simulink model "air_m0c"  (R2022b)
settings: Solver=FixedStepAuto  StartTime=0.0  StopTime=10.0  FixedStep=0.001  RelTol=1e-3  EnableMultiTasking=on
values from neighbouring files (symbols this model uses):
  dev = abs(cand(k) - cand(k - 1))    [m3_check_execution.m]
undefined symbols (not defined in the file or in its folder): Main, pwm_output0
libraries: simulink x1, px4lib x1, px4Sensorslib x1, shared6dof x1, sharedtransform x1
settings Model: ExtModeTrigDuration=10  Creator=admin  LastModifiedBy=10444
settings SolverCC: AlgebraicLoopSolver=TrustRegion  PositivePriorityOrder=on  AutoInsertRateTranBlk=on  MaxZcPerStep=1
settings OptimizationCC: EnhancedBackFolding=on  PassReuseOutputArgsAs=Individual arguments  ZeroExternalMemoryAtStartup=off  ZeroInternalMemoryAtStartup=off  MaxStackSize=64  OptimizeBlockOrder=speed  DifferentSizesBufferReuse=on  OptimizationCustomize=off  EfficientTunableParamExpr=on
settings DebuggingCC: ParameterTunabilityLossMsg=error  UnconnectedInputMsg=warning  UnconnectedOutputMsg=warning  UnconnectedLineMsg=warning  SymbolicDimsDataTypeCodeGenerationDiagnostic=none  SFMachineParentedDataDiag=warning
settings HardwareCC: ProdBitPerPointer=32  ProdBitPerSizeT=32  ProdBitPerPtrDiffT=32  ProdLargestAtomicInteger=Long  ProdLargestAtomicFloat=Double  ProdWordSize=32  ProdLongLongMode=on  ProdHWDeviceType=ARM Compatible->ARM Cortex
settings ModelReferenceCC: EnableRefExpFcnMdlSchedulingChecks=on
settings SFSimCC: MATLABDynamicMemAlloc=off  SimTargetLang=C++
settings RTWCC: Description=Embedded Coder  SystemTargetFile=ert.tlc  HardwareBoard=PX4 Pixhawk 4  TLCOptions="-aInlineSetEventsForThisBaseRateFcn=TLC_FALSE -aSuppressMultiTaskScheduler=TLC_FALSE  -aRateBasedStepFcn=0"  TemplateMakefile=ert_default_tmf  Toolchain=GNU Tools for PX4 Autopilots  IncludeHyperlinkInReport=on  TargetLang=C++  DLArmComputeVersion=19.05
settings CodeAppCC: ForceParamTrailComments=on  IgnoreCustomStorageClasses=off  OperatorAnnotations=on  SimulinkDataObjDesc=on  SFDataObjDesc=on  InsertBlockDesc=on
settings ERTTargetCC: ExtModeTransport=3  ExtModeStaticAlloc=on  ExtModeStaticAllocSize=1024  ExtModeMexFile=ext_xcp  ExtModeIntrfLevel=Level2 - Open

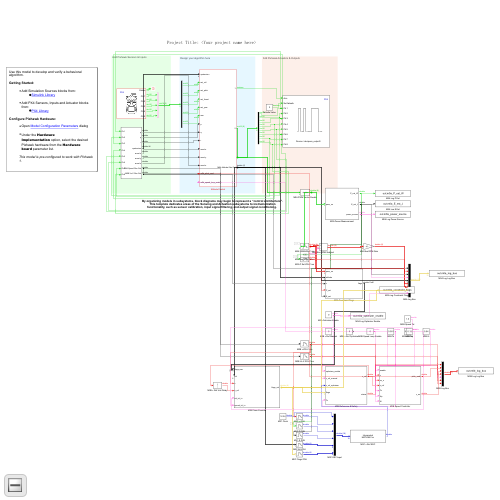
[thumbnail: Simulink's stored preview of the top-level diagram]
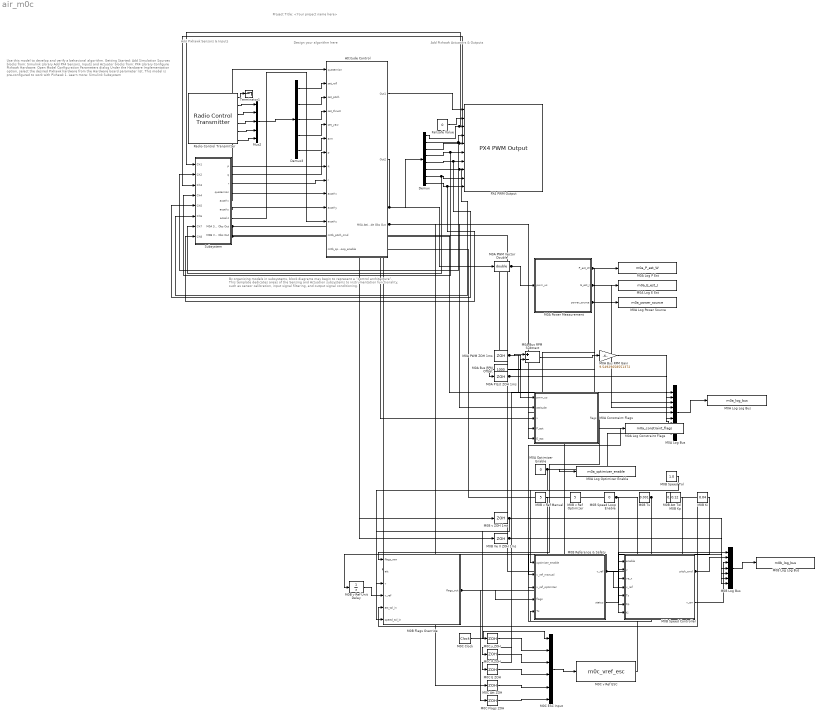
== system air_m0c ==
  note: Project Title: <Your project name here>
  note: Use this model to develop and verify a behavioral algorithm.
      |
      | Getting Started:
      |
      | Add Simulation Sources blocks from:
      | Simulink Library
      |
      | Add PX4 Sensors, Inputs and Actuator blocks from:
      | PX4 Library
      |
      | Configure Pixhawk Hardware:
      |
      | Open Model Configuration Parameters dialog
      |
      | Under the Hardware Implementation option, select the desired Pixhawk hardware from the Hardware board parameter list.
      |
      | This model is pre-configured to work with Pixhawk 1.
      |
      | Learn more:
      |
      | Simulink Subsystem
  note: Add Pixhawk Sensors & Inputs
  note: Design your algorithm here
  note: Add Pixhawk Actuators & Outputs
  note: By organizing models in subsystems, block diagrams may begin to represent a “control architecture”.
      | This template dedicates areas of the Sensing and Actuation subsystems to instrumentation functionality, such as sensor calibration, input signal filtering, and output signal conditioning.
  Attitude Control : Subsystem
  Demux : Demux  Outputs=8
  Demux3 : Demux  Outputs=5
  Failsafe Value : Constant  Value=0  OutDataTypeStr=boolean  SampleTime=-1
  M0A Bus RPM Gain : Gain  Gain=9.54929658551372
  M0A Bus RPM Offset : Constant  Value=1000
  M0A Bus RPM Subtract : Sum  Inputs=+-
  M0A Constraint Flags : Subsystem
  M0A Log Bus : Mux  Inputs=9
  M0A Log Constraint Flags : ToWorkspace  VariableName=m0a_constraint_flags  SaveFormat=Timeseries  SampleTime=-1
  M0A Log E Est : ToWorkspace  VariableName=m0a_E_est_J  SaveFormat=Timeseries  SampleTime=-1
  M0A Log Log Bus : ToWorkspace  VariableName=m0a_log_bus  SaveFormat=Timeseries  SampleTime=-1
  M0A Log Optimizer Enable : ToWorkspace  VariableName=m0a_optimizer_enable  SaveFormat=Timeseries  SampleTime=-1
  M0A Log P Est : ToWorkspace  VariableName=m0a_P_est_W  SaveFormat=Timeseries  SampleTime=-1
  M0A Log Power Source : ToWorkspace  VariableName=m0a_power_source  SaveFormat=Timeseries  SampleTime=-1
  M0A Optimizer Enable : Constant  Value=0
  M0A P Est ZOH 1ms : ZeroOrderHold  SampleTime=0.001
  M0A PWM Vector Double : DataTypeConversion  OutDataTypeStr=double  SaturateOnIntegerOverflow=off  RndMeth=Floor
  M0A PWM ZOH 1ms : ZeroOrderHold  SampleTime=0.001
  M0A Power Measurement : Subsystem
  M0B Att Tol : Constant  Value=0.523
  M0B Flags Override : Subsystem
  M0B Ki : Constant  Value=0.04
  M0B Kp : Constant  Value=0.12
  M0B Log Bus : Mux  Inputs=7
  M0B Log Log Bus : ToWorkspace  VariableName=m0b_log_bus  SaveFormat=Timeseries  SampleTime=-1
  M0B Reference & Safety : Subsystem
  M0B Speed Controller : Subsystem
  M0B Speed Loop Enable : Constant  Value=0
  M0B Speed Tol : Constant  Value=1.0
  M0B Ts : Constant  Value=0.001
  M0B Ve X ZOH 1ms : ZeroOrderHold  SampleTime=0.001
  M0B v Ref Manual : Constant  Value=5
  M0B v Ref Optimizer : Constant  Value=5
  M0B v Ref Unit Delay : UnitDelay  SampleTime=0.001  HasFrameUpgradeWarning=on
  M0B v ZOH 1ms : ZeroOrderHold  SampleTime=0.001
  M0C Att ZOH : ZeroOrderHold  SampleTime=0.05
  M0C Clock : DigitalClock  SampleTime=0.05
  M0C E ZOH : ZeroOrderHold  SampleTime=0.05
  M0C ESC Input : Mux  Inputs=6
  M0C Flags ZOH : ZeroOrderHold  SampleTime=0.05
  M0C P ZOH : ZeroOrderHold  SampleTime=0.05
  M0C v Ref ESC : MATLABFcn  MATLABFcn=m0c_vref_esc  SampleTime=0.05
  M0C v ZOH : ZeroOrderHold  SampleTime=0.05
  Mux2 : Mux  Inputs=5
  PX4 PWM Output : px4lib/PX4 PWM Output  pwmDevice=Main (/dev/pwm_output0)  pwmChannel1_=on  pwmChannel2_=on  pwmChannel3_=on  pwmChannel4_=on  pwmChannel5_=on  pwmChannel6_=on  pwmChannel7_=on  pwmChannel8_=on  forceTerminateFailsafe=off  outputErrorStatus=off
  Radio Control Transmitter : px4Sensorslib/Radio Control Transmitter  channel1=on  channel2=on  channel3=on  channel4=on  channel5=on  channel6=off  channel7=off  channel8=off  channel_count=off  rssi=off  rc_input_source=off  timestamp_last_signal=off  time_stamp=off  sampleTime=1/250  BlockingMode=off  BlockTimeout=5
  Subsystem : Subsystem
  Terminator1 : Terminator
  wires:
  Radio Control Transmitter/1 -> Terminator1/1
  Failsafe Value/1 -> PX4 PWM Output/2
  Attitude Control/1(Out1) -> PX4 PWM Output/1
  Attitude Control/2(Out2) -> Demux/1, M0A PWM Vector Double/1
  Demux/4 -> Subsystem/4(Ch4), PX4 PWM Output/6
  Demux/3 -> Subsystem/3(Ch3), PX4 PWM Output/5
  Demux/2 -> Subsystem/2(Ch2), PX4 PWM Output/4
  Demux/1 -> PX4 PWM Output/3, Subsystem/1(Ch1)
  Mux2/1 -> Demux3/1
  Radio Control Transmitter/2 -> Mux2/1
  Radio Control Transmitter/3 -> Mux2/2
  Radio Control Transmitter/4 -> Mux2/3
  Radio Control Transmitter/5 -> Mux2/4
  Radio Control Transmitter/6 -> Mux2/5
  Demux3/2 -> Attitude Control/3(set_pitch)
  Demux3/3 -> Attitude Control/4(set_thrust)
  Demux3/1 -> Attitude Control/2(set_roll)
  Demux3/4 -> Attitude Control/5(set_yaw)
  Demux3/5 -> Attitude Control/6(arm)
  Demux/5 -> Subsystem/5(Ch5), PX4 PWM Output/7
  Demux/6 -> Subsystem/6(Ch6), PX4 PWM Output/8
  Demux/7 -> Subsystem/7(Ch7), PX4 PWM Output/9
  Demux/8 -> Subsystem/8(Ch8), PX4 PWM Output/10
  Subsystem/1(p) -> Attitude Control/7(p)
  Subsystem/2(q) -> Attitude Control/8(q)
  Subsystem/3(r) -> Attitude Control/9(r)
  Subsystem/4(quaternion) -> Attitude Control/1(quaternion)
  Subsystem/5(accel-x) -> Attitude Control/10(accel-x)
  Subsystem/6(accel-y) -> Attitude Control/11(accel-y)
  Subsystem/7(accel-z) -> Attitude Control/12(accel-z)
  M0A PWM Vector Double/1 -> M0A Power Measurement/1(pwm_us), M0A PWM ZOH 1ms/1
  M0A Power Measurement/1(P_est_W) -> M0A Log P Est/1, M0A P Est ZOH 1ms/1, M0C P ZOH/1
  M0A Power Measurement/2(E_est_J) -> M0A Log E Est/1, M0A Constraint Flags/5(E_est), M0A Log Bus/3, M0C E ZOH/1
  M0A Power Measurement/3(power_source) -> M0A Log Power Source/1, M0A Log Bus/4
  M0A PWM ZOH 1ms/1 -> M0A Constraint Flags/1(pwm_us), M0A Log Bus/6, M0A Bus RPM Subtract/1
  Attitude Control/3(M0A Attitude Obs Out) -> M0A Constraint Flags/2(attitude), M0A Log Bus/5, M0B Flags Override/2(att), M0C Att ZOH/1
  Subsystem/8(M0A Speed Obs Out) -> M0A Constraint Flags/3(v), M0A Log Bus/1, M0B v ZOH 1ms/1
  M0A P Est ZOH 1ms/1 -> M0A Constraint Flags/4(P_est), M0A Log Bus/2
  M0A Constraint Flags/1(flags) -> M0B Flags Override/1(flags_raw)
  M0A Optimizer Enable/1 -> M0A Log Bus/9, M0A Log Optimizer Enable/1, M0B Reference & Safety/1(optimizer_enable)
  M0A Log Bus/1 -> M0A Log Log Bus/1
  M0A Bus RPM Offset/1 -> M0A Bus RPM Subtract/2
  M0A Bus RPM Subtract/1 -> M0A Bus RPM Gain/1
  M0A Bus RPM Gain/1 -> M0A Log Bus/7
  Subsystem/9(M0B Ve X Obs Out) -> M0B Ve X ZOH 1ms/1
  M0B v Ref Manual/1 -> M0B Reference & Safety/2(v_ref_manual)
  M0B Ts/1 -> M0B Reference & Safety/5(Ts), M0B Speed Controller/5(Ts)
  M0B Speed Loop Enable/1 -> M0B Speed Controller/1(enable), Attitude Control/14(m0b_speed_loop_enable), M0B Log Bus/5
  M0B v ZOH 1ms/1 -> M0B Speed Controller/2(v), M0B Flags Override/3(v), M0B Log Bus/7, M0C v ZOH/1
  M0B Ve X ZOH 1ms/1 -> M0B Speed Controller/3(ve_x), M0B Log Bus/6
  M0B Reference & Safety/1(v_ref) -> M0B Speed Controller/4(v_ref), M0B v Ref Unit Delay/1, M0B Log Bus/1
  M0B Speed Controller/1(pitch_cmd) -> Attitude Control/13(m0b_pitch_cmd), M0B Log Bus/2
  M0B v Ref Unit Delay/1 -> M0B Flags Override/4(v_ref)
  M0B Att Tol/1 -> M0B Flags Override/5(att_tol_in)
  M0B Speed Tol/1 -> M0B Flags Override/6(speed_tol_in)
  M0B Speed Controller/2(v_err) -> M0B Log Bus/3
  M0B Reference & Safety/2(status) -> M0B Log Bus/4
  M0B Log Bus/1 -> M0B Log Log Bus/1
  M0B Flags Override/1(flags_out) -> M0A Log Bus/8, M0B Reference & Safety/4(flags), M0A Log Constraint Flags/1, M0C Flags ZOH/1
  M0B Kp/1 -> M0B Speed Controller/6(Kp)
  M0B Ki/1 -> M0B Speed Controller/7(Ki)
  M0C v ZOH/1 -> M0C ESC Input/2
  M0C P ZOH/1 -> M0C ESC Input/3
  M0C E ZOH/1 -> M0C ESC Input/4
  M0C Att ZOH/1 -> M0C ESC Input/5
  M0C Flags ZOH/1 -> M0C ESC Input/6
  M0C Clock/1 -> M0C ESC Input/1
  M0C ESC Input/1 -> M0C v Ref ESC/1
  M0C v Ref ESC/1 -> M0B Reference & Safety/3(v_ref_optimizer)

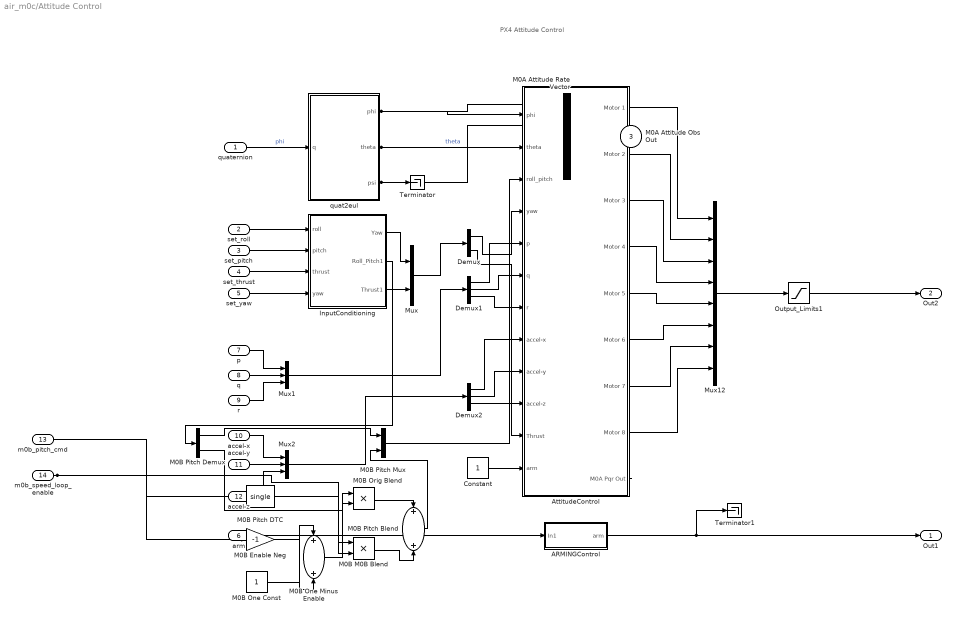
== system air_m0c/Attitude Control ==
  note: PX4 Attitude Control
  quaternion : Inport
  set_roll : Inport  Port=2  OutDataTypeStr=uint16
  set_pitch : Inport  Port=3  OutDataTypeStr=uint16
  set_thrust : Inport  Port=4  OutDataTypeStr=uint16
  set_yaw : Inport  Port=5  OutDataTypeStr=uint16
  arm : Inport  Port=6  OutDataTypeStr=uint16
  p : Inport  Port=7
  q : Inport  Port=8
  r : Inport  Port=9
  accel-x : Inport  Port=10
  accel-y : Inport  Port=11
  accel-z : Inport  Port=12
  m0b_pitch_cmd : Inport  Port=13
  m0b_speed_loop_enable : Inport  Port=14
  ARMINGControl : Subsystem
  AttitudeControl : Subsystem
  Constant : Constant
  Demux : Demux  Outputs=2
  Demux1 : Demux  Outputs=3
  Demux2 : Demux  Outputs=3
  InputConditioning : Subsystem
  M0A Attitude Rate Vector : Mux
  M0B Enable Neg : Gain  Gain=-1
  M0B M0B Blend : Product
  M0B One Const : Constant
  M0B One Minus Enable : Sum
  M0B Orig Blend : Product
  M0B Pitch Blend : Sum
  M0B Pitch DTC : DataTypeConversion  OutDataTypeStr=single  SaturateOnIntegerOverflow=off  RndMeth=Floor
  M0B Pitch Demux : Demux  Outputs=2
  M0B Pitch Mux : Mux  Inputs=2
  Mux : Mux  Inputs=2
  Mux1 : Mux  Inputs=3
  Mux12 : Mux  Inputs=8
  Mux2 : Mux  Inputs=3
  Output_Limits1 : Saturate  UpperLimit=2000  LowerLimit=1000
  Terminator : Terminator
  Terminator1 : Terminator
  quat2eul : MATLAB Function  TreatAsAtomicUnit=on
  Out1 : Outport  VectorParamsAs1DForOutWhenUnconnected=off
  Out2 : Outport  Port=2  VectorParamsAs1DForOutWhenUnconnected=off
  M0A Attitude Obs Out : Outport  Port=3
  wires:
  set_pitch/1 -> InputConditioning/2(pitch)
  set_roll/1 -> InputConditioning/1(roll)
  quat2eul/2(theta) -> AttitudeControl/2(theta), M0A Attitude Rate Vector/2  "theta"
  Output_Limits1/1 -> Out2/1
  set_thrust/1 -> InputConditioning/3(thrust)
  Mux12/1 -> Output_Limits1/1
  ARMINGControl/1(arm) -> Terminator1/1, Out1/1
  set_yaw/1 -> InputConditioning/4(yaw)
  quaternion/1 -> quat2eul/1(q)  "phi"
  quat2eul/1(phi) -> AttitudeControl/1(phi), M0A Attitude Rate Vector/1
  quat2eul/3(psi) -> Terminator/1, M0A Attitude Rate Vector/3
  AttitudeControl/1(Motor 1) -> Mux12/1
  AttitudeControl/2(Motor 2) -> Mux12/2
  AttitudeControl/3(Motor 3) -> Mux12/3
  Mux/1 -> Demux/1
  q/1 -> Mux1/2
  p/1 -> Mux1/1
  r/1 -> Mux1/3
  Mux1/1 -> Demux1/1
  Demux1/2 -> AttitudeControl/6(q)
  Demux1/1 -> AttitudeControl/5(p)
  Demux1/3 -> AttitudeControl/7(r)
  accel-y/1 -> Mux2/2
  accel-x/1 -> Mux2/1
  accel-z/1 -> Mux2/3
  Mux2/1 -> Demux2/1
  Demux2/2 -> AttitudeControl/9(accel-y)
  Demux2/1 -> AttitudeControl/8(accel-x)
  Demux2/3 -> AttitudeControl/10(accel-z)
  InputConditioning/1(Yaw) -> Mux/1
  Demux/1 -> AttitudeControl/4(yaw)
  Demux/2 -> AttitudeControl/11(Thrust)
  AttitudeControl/4(Motor 4) -> Mux12/4
  AttitudeControl/5(Motor 5) -> Mux12/5
  AttitudeControl/6(Motor 6) -> Mux12/6
  AttitudeControl/7(Motor 7) -> Mux12/7
  AttitudeControl/8(Motor 8) -> Mux12/8
  Constant/1 -> AttitudeControl/12(arm)
  InputConditioning/3(Thrust1) -> Mux/2
  arm/1 -> ARMINGControl/1(In1)
  AttitudeControl/9(M0A Pqr Out) -> M0A Attitude Rate Vector/4
  M0A Attitude Rate Vector/1 -> M0A Attitude Obs Out/1
  InputConditioning/2(Roll_Pitch1) -> M0B Pitch Demux/1
  M0B Pitch Demux/1 -> M0B Pitch Mux/1
  M0B Pitch Demux/2 -> M0B Orig Blend/1
  m0b_speed_loop_enable/1 -> M0B Enable Neg/1, M0B M0B Blend/2
  M0B One Const/1 -> M0B One Minus Enable/1
  M0B Enable Neg/1 -> M0B One Minus Enable/2
  M0B One Minus Enable/1 -> M0B Orig Blend/2
  m0b_pitch_cmd/1 -> M0B Pitch DTC/1
  M0B Pitch DTC/1 -> M0B M0B Blend/1
  M0B Orig Blend/1 -> M0B Pitch Blend/1
  M0B M0B Blend/1 -> M0B Pitch Blend/2
  M0B Pitch Blend/1 -> M0B Pitch Mux/2
  M0B Pitch Mux/1 -> AttitudeControl/3(roll_pitch)

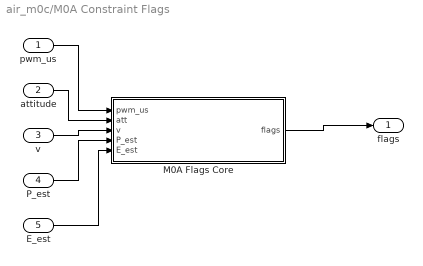
== system air_m0c/M0A Constraint Flags ==
  pwm_us : Inport
  attitude : Inport  Port=2
  v : Inport  Port=3
  P_est : Inport  Port=4
  E_est : Inport  Port=5
  M0A Flags Core : MATLAB Function  TreatAsAtomicUnit=on
  flags : Outport
  wires:
  pwm_us/1 -> M0A Flags Core/1(pwm_us)
  attitude/1 -> M0A Flags Core/2(att)
  v/1 -> M0A Flags Core/3(v)
  P_est/1 -> M0A Flags Core/4(P_est)
  E_est/1 -> M0A Flags Core/5(E_est)
  M0A Flags Core/1(flags) -> flags/1

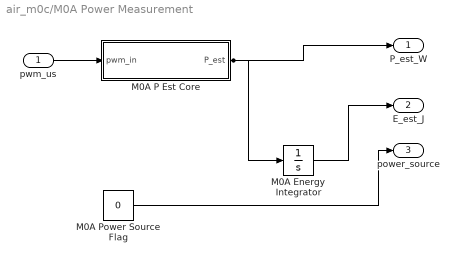
== system air_m0c/M0A Power Measurement ==
  pwm_us : Inport
  M0A Energy Integrator : Integrator
  M0A P Est Core : MATLAB Function  TreatAsAtomicUnit=on
  M0A Power Source Flag : Constant  Value=0
  P_est_W : Outport
  E_est_J : Outport  Port=2
  power_source : Outport  Port=3
  wires:
  pwm_us/1 -> M0A P Est Core/1(pwm_in)
  M0A P Est Core/1(P_est) -> M0A Energy Integrator/1, P_est_W/1
  M0A Energy Integrator/1 -> E_est_J/1
  M0A Power Source Flag/1 -> power_source/1

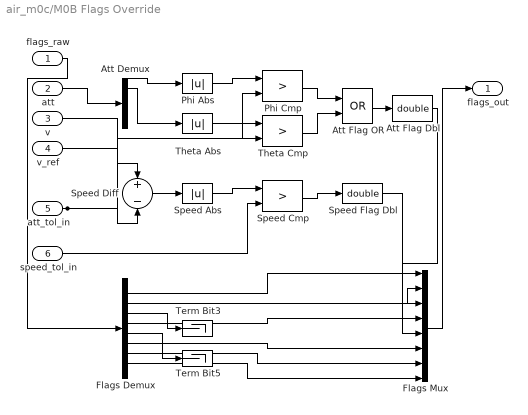
== system air_m0c/M0B Flags Override ==
  flags_raw : Inport
  att : Inport  Port=2
  v : Inport  Port=3
  v_ref : Inport  Port=4
  att_tol_in : Inport  Port=5
  speed_tol_in : Inport  Port=6
  Att Demux : Demux  Outputs=6
  Att Flag Dbl : DataTypeConversion  OutDataTypeStr=double  SaturateOnIntegerOverflow=off  RndMeth=Floor
  Att Flag OR : Logic  Operator=OR  AllPortsSameDT=off  OutDataTypeStr=boolean
  Flags Demux : Demux  Outputs=8
  Flags Mux : Mux  Inputs=8
  Phi Abs : Abs  SaturateOnIntegerOverflow=off
  Phi Cmp : RelationalOperator  Operator=>  OutDataTypeStr=boolean  RndMeth=Simplest  InputSameDT=off
  Speed Abs : Abs  SaturateOnIntegerOverflow=off
  Speed Cmp : RelationalOperator  Operator=>  OutDataTypeStr=boolean  RndMeth=Simplest  InputSameDT=off
  Speed Diff : Sum  Inputs=+-
  Speed Flag Dbl : DataTypeConversion  OutDataTypeStr=double  SaturateOnIntegerOverflow=off  RndMeth=Floor
  Term Bit3 : Terminator
  Term Bit5 : Terminator
  Theta Abs : Abs  SaturateOnIntegerOverflow=off
  Theta Cmp : RelationalOperator  Operator=>  OutDataTypeStr=boolean  RndMeth=Simplest  InputSameDT=off
  flags_out : Outport
  wires:
  att/1 -> Att Demux/1
  Att Demux/1 -> Phi Abs/1
  Att Demux/2 -> Theta Abs/1
  Phi Abs/1 -> Phi Cmp/1
  Theta Abs/1 -> Theta Cmp/1
  att_tol_in/1 -> Phi Cmp/2, Theta Cmp/2
  Phi Cmp/1 -> Att Flag OR/1
  Theta Cmp/1 -> Att Flag OR/2
  Att Flag OR/1 -> Att Flag Dbl/1
  v/1 -> Speed Diff/1
  v_ref/1 -> Speed Diff/2
  Speed Diff/1 -> Speed Abs/1
  Speed Abs/1 -> Speed Cmp/1
  speed_tol_in/1 -> Speed Cmp/2
  Speed Cmp/1 -> Speed Flag Dbl/1
  flags_raw/1 -> Flags Demux/1
  Flags Demux/1 -> Flags Mux/1
  Flags Demux/2 -> Flags Mux/2
  Att Flag Dbl/1 -> Flags Mux/3
  Flags Demux/4 -> Flags Mux/4
  Speed Flag Dbl/1 -> Flags Mux/5
  Flags Demux/6 -> Flags Mux/6
  Flags Demux/7 -> Flags Mux/7
  Flags Demux/8 -> Flags Mux/8
  Flags Mux/1 -> flags_out/1
  Flags Demux/3 -> Term Bit3/1
  Flags Demux/5 -> Term Bit5/1

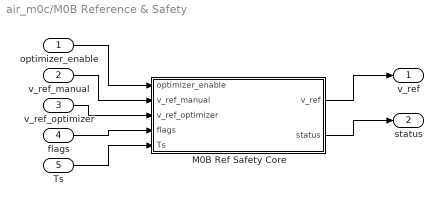
== system air_m0c/M0B Reference & Safety ==
  optimizer_enable : Inport
  v_ref_manual : Inport  Port=2
  v_ref_optimizer : Inport  Port=3
  flags : Inport  Port=4
  Ts : Inport  Port=5
  M0B Ref Safety Core : MATLAB Function  TreatAsAtomicUnit=on  SystemSampleTime=0.001
  v_ref : Outport
  status : Outport  Port=2
  wires:
  optimizer_enable/1 -> M0B Ref Safety Core/1(optimizer_enable)
  v_ref_manual/1 -> M0B Ref Safety Core/2(v_ref_manual)
  v_ref_optimizer/1 -> M0B Ref Safety Core/3(v_ref_optimizer)
  flags/1 -> M0B Ref Safety Core/4(flags)
  Ts/1 -> M0B Ref Safety Core/5(Ts)
  M0B Ref Safety Core/1(v_ref) -> v_ref/1
  M0B Ref Safety Core/2(status) -> status/1

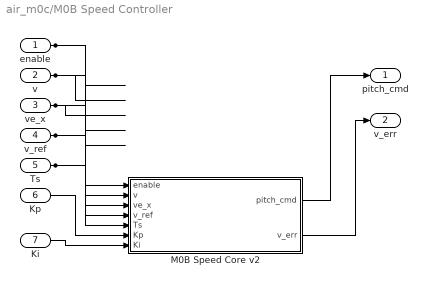
== system air_m0c/M0B Speed Controller ==
  enable : Inport
  v : Inport  Port=2
  ve_x : Inport  Port=3
  v_ref : Inport  Port=4
  Ts : Inport  Port=5
  Kp : Inport  Port=6
  Ki : Inport  Port=7
  M0B Speed Core v2 : MATLAB Function  TreatAsAtomicUnit=on  SystemSampleTime=0.001
  pitch_cmd : Outport
  v_err : Outport  Port=2
  wires:
  enable/1 -> M0B Speed Core v2/1(enable)
  v/1 -> M0B Speed Core v2/2(v)
  ve_x/1 -> M0B Speed Core v2/3(ve_x)
  v_ref/1 -> M0B Speed Core v2/4(v_ref)
  Ts/1 -> M0B Speed Core v2/5(Ts)
  Kp/1 -> M0B Speed Core v2/6(Kp)
  Ki/1 -> M0B Speed Core v2/7(Ki)
  M0B Speed Core v2/1(pitch_cmd) -> pitch_cmd/1
  M0B Speed Core v2/2(v_err) -> v_err/1

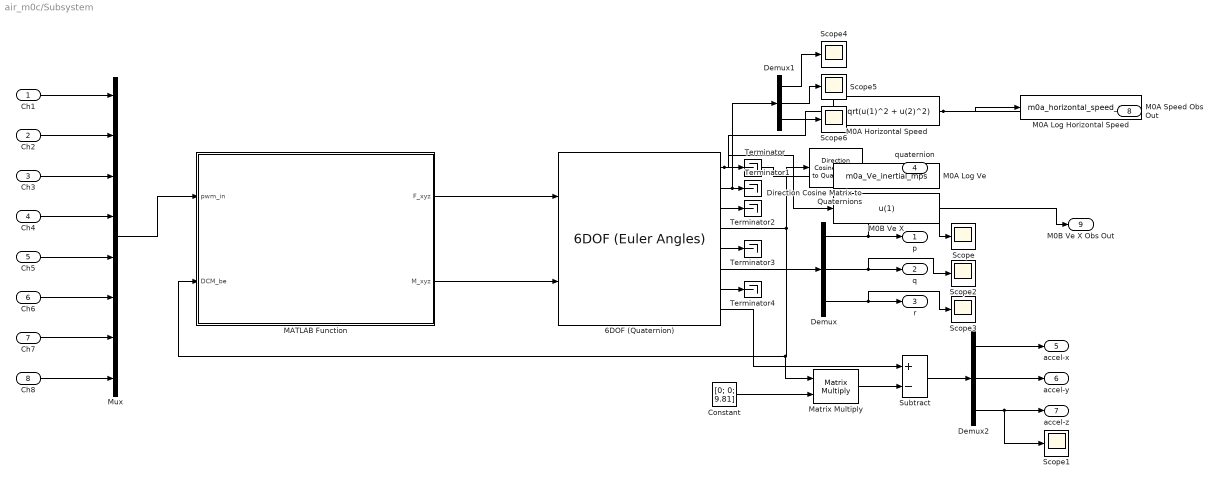
== system air_m0c/Subsystem ==
  Ch1 : Inport
  Ch2 : Inport  Port=2
  Ch3 : Inport  Port=3
  Ch4 : Inport  Port=4
  Ch5 : Inport  Port=5
  Ch6 : Inport  Port=6
  Ch7 : Inport  Port=7
  Ch8 : Inport  Port=8
  6DOF (Quaternion) : shared6dof/6DOF (Euler Angles)  units=Metric (MKS)  mtype=Fixed  rep=Quaternion  xme_0=[0 0 0]  Vm_0=[0 0 0]  eul_0=[0 0 0]  pm_0=[0 0 0]  mass_0=1.4  mass_e=0.5  mass_f=2.0  inertia=diag([0.0165, 0.0165, 0.0292])  inertia_e=eye(3)  inertia_f=2*eye(3)  k_quat=1.0  vre_flag=on  abi_flag=off  aMode=0  xme_statename=''  Vm_statename=''  eul_statename=''  quat_statename=''  pm_statename=''  mass_statename=''
      settings: LibrarySourceBlock=aerolib6dof2/6DOF (Quaternion)
  Constant : Constant  Value=[0; 0; 9.81]
  Demux : Demux  Outputs=3
  Demux1 : Demux  Outputs=3
  Demux2 : Demux  Outputs=3
  Direction Cosine Matrix to Quaternions : sharedtransform/Direction Cosine Matrix  to Quaternions  aMode=0  action=None  tolerance=eps(2)
      settings: LibrarySourceBlock=|
      | aerolibtransform2/Direction Cosine Matrix
      | to Quaternions
  M0A Horizontal Speed : Fcn  Expr=sqrt(u(1)^2 + u(2)^2)
  M0A Log Horizontal Speed : ToWorkspace  VariableName=m0a_horizontal_speed_mps  SaveFormat=Timeseries  SampleTime=-1
  M0A Log Ve : ToWorkspace  VariableName=m0a_Ve_inertial_mps  SaveFormat=Timeseries  SampleTime=-1
  M0B Ve X : Fcn  Expr=u(1)
  MATLAB Function : MATLAB Function  TreatAsAtomicUnit=on
  Matrix Multiply : Product  Multiplication=Matrix(*)
  Mux : Mux  Inputs=8
  Scope{,1..6} (7 alike) : Scope
  Subtract : Sum  Inputs=+-
  Terminator{,1..4} (5 alike) : Terminator
  p : Outport
  q : Outport  Port=2
  r : Outport  Port=3
  quaternion : Outport  Port=4
  accel-x : Outport  Port=5
  accel-y : Outport  Port=6
  accel-z : Outport  Port=7
  M0A Speed Obs Out : Outport  Port=8
  M0B Ve X Obs Out : Outport  Port=9
  wires:
  6DOF (Quaternion)/5 -> Terminator3/1
  Demux/2 -> Scope2/1, q/1
  Ch5/1 -> Mux/5
  Mux/1 -> MATLAB Function/1(pwm_in)
  Constant/1 -> Matrix Multiply/2
  Ch2/1 -> Mux/2
  6DOF (Quaternion)/3 -> Terminator2/1
  Ch4/1 -> Mux/4
  MATLAB Function/1(F_xyz) -> 6DOF (Quaternion)/1
  MATLAB Function/2(M_xyz) -> 6DOF (Quaternion)/2
  Matrix Multiply/1 -> Subtract/2
  Demux/1 -> Scope/1, p/1
  Demux2/3 -> accel-z/1, Scope1/1
  Demux/3 -> Scope3/1, r/1
  6DOF (Quaternion)/4 -> Direction Cosine Matrix to Quaternions/1, Matrix Multiply/1, MATLAB Function/2(DCM_be)
  Subtract/1 -> Demux2/1
  6DOF (Quaternion)/6 -> Demux/1
  Ch3/1 -> Mux/3
  6DOF (Quaternion)/7 -> Terminator4/1
  Demux2/2 -> accel-y/1
  6DOF (Quaternion)/2 -> Demux1/1, Terminator1/1
  Direction Cosine Matrix to Quaternions/1 -> quaternion/1
  Ch1/1 -> Mux/1
  Ch7/1 -> Mux/7
  6DOF (Quaternion)/8 -> Subtract/1
  Ch6/1 -> Mux/6
  Demux2/1 -> accel-x/1
  6DOF (Quaternion)/1 -> Terminator/1, M0A Horizontal Speed/1, M0A Log Ve/1, M0B Ve X/1
  Ch8/1 -> Mux/8
  Demux1/1 -> Scope4/1
  Demux1/2 -> Scope5/1
  Demux1/3 -> Scope6/1
  M0A Horizontal Speed/1 -> M0A Log Horizontal Speed/1, M0A Speed Obs Out/1
  M0B Ve X/1 -> M0B Ve X Obs Out/1

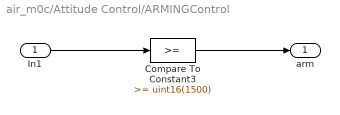
== system air_m0c/Attitude Control/ARMINGControl ==
  In1 : Inport
  Compare To Constant3 : simulink/Logic and Bit Operations/Compare To Constant  relop=>=  const=uint16(1500)  OutDataTypeStr=boolean
  arm : Outport  VectorParamsAs1DForOutWhenUnconnected=off
  wires:
  Compare To Constant3/1 -> arm/1
  In1/1 -> Compare To Constant3/1

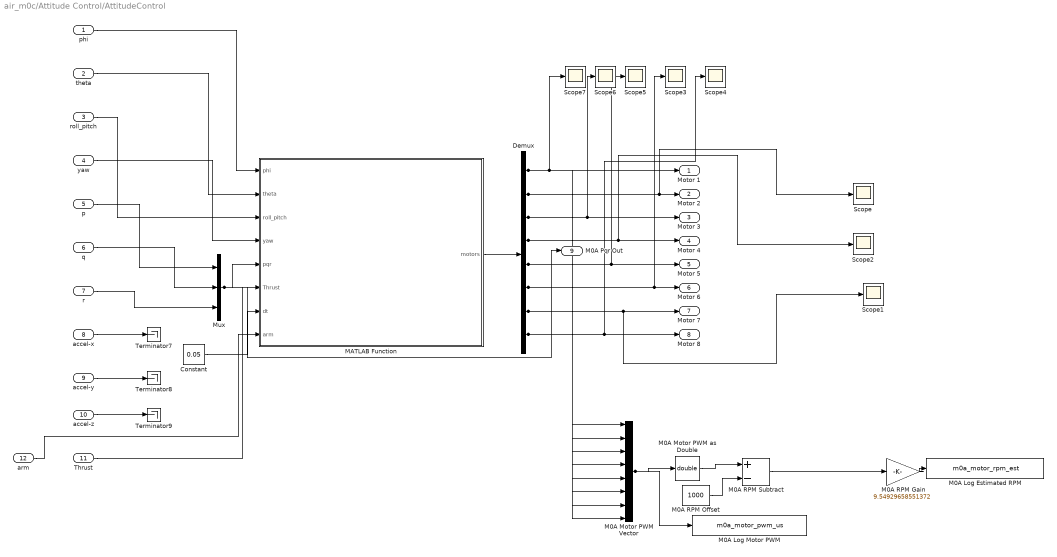
== system air_m0c/Attitude Control/AttitudeControl ==
  phi : Inport
  theta : Inport  Port=2
  roll_pitch : Inport  Port=3
  yaw : Inport  Port=4
  p : Inport  Port=5
  q : Inport  Port=6
  r : Inport  Port=7
  accel-x : Inport  Port=8
  accel-y : Inport  Port=9
  accel-z : Inport  Port=10
  Thrust : Inport  Port=11
  arm : Inport  Port=12
  Constant : Constant  Value=0.05
  Demux : Demux  Outputs=8
  M0A Log Estimated RPM : ToWorkspace  VariableName=m0a_motor_rpm_est  SaveFormat=Timeseries  SampleTime=-1
  M0A Log Motor PWM : ToWorkspace  VariableName=m0a_motor_pwm_us  SaveFormat=Timeseries  SampleTime=-1
  M0A Motor PWM Vector : Mux  Inputs=8
  M0A Motor PWM as Double : DataTypeConversion  OutDataTypeStr=double  SaturateOnIntegerOverflow=off  RndMeth=Floor
  M0A RPM Gain : Gain  Gain=9.54929658551372
  M0A RPM Offset : Constant  Value=1000
  M0A RPM Subtract : Sum  Inputs=+-
  MATLAB Function : MATLAB Function  TreatAsAtomicUnit=on
  Mux : Mux  Inputs=3
  Scope{,1..7} (8 alike) : Scope
  Terminator7 : Terminator
  Terminator8 : Terminator
  Terminator9 : Terminator
  Motor 1 : Outport  OutDataTypeStr=uint16  SampleTime=1/250  VectorParamsAs1DForOutWhenUnconnected=off
  Motor 2 : Outport  Port=2  OutDataTypeStr=uint16  SampleTime=1/250  VectorParamsAs1DForOutWhenUnconnected=off
  Motor 3 : Outport  Port=3  OutDataTypeStr=uint16  SampleTime=1/250  VectorParamsAs1DForOutWhenUnconnected=off
  Motor 4 : Outport  Port=4  OutDataTypeStr=uint16  SampleTime=1/250  VectorParamsAs1DForOutWhenUnconnected=off
  Motor 5 : Outport  Port=5  OutDataTypeStr=uint16  SampleTime=1/250  VectorParamsAs1DForOutWhenUnconnected=off
  Motor 6 : Outport  Port=6  OutDataTypeStr=uint16  SampleTime=1/250  VectorParamsAs1DForOutWhenUnconnected=off
  Motor 7 : Outport  Port=7  OutDataTypeStr=uint16  SampleTime=1/250  VectorParamsAs1DForOutWhenUnconnected=off
  Motor 8 : Outport  Port=8  OutDataTypeStr=uint16  SampleTime=1/250  VectorParamsAs1DForOutWhenUnconnected=off
  M0A Pqr Out : Outport  Port=9
  wires:
  roll_pitch/1 -> MATLAB Function/3(roll_pitch)
  p/1 -> Mux/1
  accel-x/1 -> Terminator7/1
  accel-y/1 -> Terminator8/1
  accel-z/1 -> Terminator9/1
  Thrust/1 -> MATLAB Function/6(Thrust)
  q/1 -> Mux/2
  r/1 -> Mux/3
  Mux/1 -> MATLAB Function/5(pqr), M0A Pqr Out/1
  Constant/1 -> MATLAB Function/7(dt)
  MATLAB Function/1(motors) -> Demux/1
  Demux/1 -> Motor 1/1, Scope7/1, M0A Motor PWM Vector/1
  Demux/2 -> Scope/1, Motor 2/1, M0A Motor PWM Vector/2
  Demux/3 -> Scope6/1, Motor 3/1, M0A Motor PWM Vector/3
  Demux/4 -> Scope2/1, Motor 4/1, M0A Motor PWM Vector/4
  Demux/5 -> Motor 5/1, Scope5/1, M0A Motor PWM Vector/5
  Demux/6 -> Scope3/1, Motor 6/1, M0A Motor PWM Vector/6
  Demux/7 -> Scope1/1, Motor 7/1, M0A Motor PWM Vector/7
  Demux/8 -> Scope4/1, Motor 8/1, M0A Motor PWM Vector/8
  phi/1 -> MATLAB Function/1(phi)
  theta/1 -> MATLAB Function/2(theta)
  yaw/1 -> MATLAB Function/4(yaw)
  arm/1 -> MATLAB Function/8(arm)
  M0A Motor PWM Vector/1 -> M0A Motor PWM as Double/1, M0A Log Motor PWM/1
  M0A Motor PWM as Double/1 -> M0A RPM Subtract/1
  M0A RPM Offset/1 -> M0A RPM Subtract/2
  M0A RPM Subtract/1 -> M0A RPM Gain/1
  M0A RPM Gain/1 -> M0A Log Estimated RPM/1

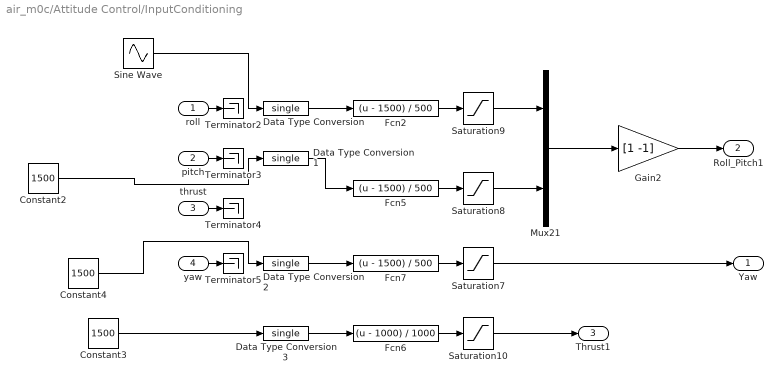
== system air_m0c/Attitude Control/InputConditioning ==
  roll : Inport
  pitch : Inport  Port=2
  thrust : Inport  Port=3
  yaw : Inport  Port=4
  Constant2 : Constant  Value=1500
  Constant3 : Constant  Value=1500
  Constant4 : Constant  Value=1500
  Data Type Conversion{,1..3} (4 alike) : DataTypeConversion  OutDataTypeStr=single  SaturateOnIntegerOverflow=off  RndMeth=Floor
  Fcn2 : Fcn  Expr=(u - 1500) / 500
  Fcn5 : Fcn  Expr=(u - 1500) / 500
  Fcn6 : Fcn  Expr=(u - 1000) / 1000
  Fcn7 : Fcn  Expr=(u - 1500) / 500
  Gain2 : Gain  Gain=[1 -1]  OutDataTypeStr=Inherit: Inherit via back propagation
  Mux21 : Mux  Inputs=2
  Saturation10 : Saturate  UpperLimit=1  LowerLimit=0
  Saturation7 : Saturate  UpperLimit=1  LowerLimit=-1
  Saturation8 : Saturate  UpperLimit=1  LowerLimit=-1
  Saturation9 : Saturate  UpperLimit=1  LowerLimit=-1
  Sine Wave : Sin  Amplitude=200  Bias=1500  SampleTime=0
  Terminator{2..5} (4 alike) : Terminator
  Yaw : Outport  VectorParamsAs1DForOutWhenUnconnected=off
  Roll_Pitch1 : Outport  Port=2  VectorParamsAs1DForOutWhenUnconnected=off
  Thrust1 : Outport  Port=3  VectorParamsAs1DForOutWhenUnconnected=off
  wires:
  Saturation10/1 -> Thrust1/1
  Saturation7/1 -> Yaw/1
  Gain2/1 -> Roll_Pitch1/1
  Mux21/1 -> Gain2/1
  Saturation8/1 -> Mux21/2
  Fcn6/1 -> Saturation10/1
  Fcn2/1 -> Saturation9/1
  Fcn5/1 -> Saturation8/1
  Saturation9/1 -> Mux21/1
  Fcn7/1 -> Saturation7/1
  Data Type Conversion/1 -> Fcn2/1
  Data Type Conversion1/1 -> Fcn5/1
  Data Type Conversion2/1 -> Fcn7/1
  Data Type Conversion3/1 -> Fcn6/1
  roll/1 -> Terminator2/1
  pitch/1 -> Terminator3/1
  thrust/1 -> Terminator4/1
  yaw/1 -> Terminator5/1
  Constant2/1 -> Data Type Conversion1/1
  Constant3/1 -> Data Type Conversion3/1
  Constant4/1 -> Data Type Conversion2/1
  Sine Wave/1 -> Data Type Conversion/1

== matlab function air_m0c/Subsystem/MATLAB Function ==
  data: pwm_in input; F_xyz output; M_xyz output; DCM_be input
function [F_xyz, M_xyz] = fcn(pwm_in, DCM_be)
    % 输入: 
    %   pwm_in: 8x1 向量, [1000, 2000] us 之间的PWM信号
    %   DCM_be: 3x3 矩阵, 惯性系到机体坐标系的旋转矩阵 (Direction Cosine Matrix)
    % 输出:
    %   F_xyz:  3x1 向量, 机体坐标系下的三轴总外力 (气动力 + 重力) (N)
    %   M_xyz:  3x1 向量, 机体坐标系下的三轴总力矩 (N-m)

    %% ------------------- 1. 物理参数配置 -------------------
    m = 1.4;          % 无人机总质量 (kg)，需与 6DOF 模块中设定的质量严格一致
    g = 9.81;         % 重力加速度 (m/s^2)
    
    pwm_min   = 1000.0; 
    pwm_max   = 2000.0; 
    omega_max = 1000.0;  

    pwm_in = double(pwm_in);
    
    C_T = 1.42e-5; 
    C_M = 2.51e-7;  
    L = 0.2;       
    
    theta = [pi/4; 7*pi/4; 5*pi/4; 3*pi/4; pi/4; 7*pi/4; 5*pi/4; 3*pi/4]; 
    dir = [-1; 1; -1; 1; 1; -1; 1; -1]; 

    %% ------------------- 2. 电机动力学 -------------------
    pwm_clamped = max(min(pwm_in, pwm_max), pwm_min); 
    omega = (pwm_clamped - pwm_min) / (pwm_max - pwm_min) * omega_max; 
    
    T_i = C_T * (omega .^ 2); 
    T_i_double = double(T_i);
    Q_i = C_M * (omega .^ 2); 
    Q_i_double = double(Q_i);

    %% ------------------- 3. 力与坐标系投影计算 -------------------
    % 3.1 气动力合力计算 (机体坐标系)
    F_aero = zeros(3, 1);
    F_aero(3) = -sum(T_i); % Z轴正方向朝下，升力朝上为负
    
    % 3.2 引入重力并计算总力 (机体坐标系)
    % 惯性系（NED）下的重力矢量为 [0; 0; m*g]
    % 乘 DCM_be 将其转换至机体坐标系
    F_gravity_body = DCM_be * [0; 0; m*g]; 
    F_xyz = F_aero + F_gravity_body; 
    
    % 3.3 气动力矩合力计算 (机体坐标系)
    M_xyz = zeros(3, 1);
    M_xyz(1) = sum(-L .* sin(theta) .* T_i_double); 
    M_xyz(2) = sum( L .* cos(theta) .* T_i_double); 
    M_xyz(3) = sum(-dir .* Q_i_double);             
end

== matlab function air_m0c/Attitude Control/AttitudeControl/MATLAB Function ==
  settings: updateMethod=DISCRETE
  data: phi input; motors output; theta input; roll_pitch input; yaw input; pqr input; Thrust input; dt input; arm input
function motors = control_and_mix(phi, theta, roll_pitch, yaw, pqr, Thrust, dt, arm) 
% # 共轴双桨八轴姿态控制器与混控器 (Octa-Quad X 布局) 

    % 数据类型强制转化
    phi = double(phi); 
    theta = double(theta); 
    roll_pitch = double(roll_pitch); 
    yaw = double(yaw); 
    pqr = double(pqr); 
    Thrust = double(Thrust); 
    dt = double(dt); 
    arm = double(arm); % 引入解锁信号 (1为解锁，0为未解锁)

    % 声明 PID 状态变量
    persistent roll_int pitch_int yaw_int; 
    persistent prev_err_roll prev_err_pitch prev_err_yaw; 
    
    if isempty(roll_int) 
        roll_int = 0.0; pitch_int = 0.0; yaw_int = 0.0; 
        prev_err_roll = 0.0; prev_err_pitch = 0.0; prev_err_yaw = 0.0; 
    end

    % 核心保护 1: 如果未解锁，强制输出 1000（怠速/停转），并清除所有 PID 积分历史
    if arm < 0.5 
        roll_int = 0.0; pitch_int = 0.0; yaw_int = 0.0; 
        prev_err_roll = 0.0; prev_err_pitch = 0.0; prev_err_yaw = 0.0; 
        motors = uint16(ones(8, 1) * 1000); 
        return; 
    end

    % 核心保护 2: 防止 RC 输入为 0 时计算出极端的期望角度
    cmd_roll  = max(-1.0, min(1.0, roll_pitch(1)));
    cmd_pitch = max(-1.0, min(1.0, roll_pitch(2)));
    cmd_yaw   = max(-1.0, min(1.0, yaw));
    
    phi_des   = cmd_roll  * 0.523;
    theta_des = cmd_pitch * 0.523;
    r_des     = cmd_yaw   * 1.5;
    
    T_norm = max(0.0, min(1.0, Thrust));

    % 2. 外环角度控制器 (P)
    Kp_att_roll  = 6.5; 
    Kp_att_pitch = 6.5; 
    p_des = Kp_att_roll  * (phi_des - phi); 
    q_des = Kp_att_pitch * (theta_des - theta); 

    % 3. 内环角速度控制器 (PID)
    Kp_rate_roll  = 0.15;  Ki_rate_roll  = 0.12;  Kd_rate_roll  = 0.003; 
    Kp_rate_pitch = 0.15;  Ki_rate_pitch = 0.12;  Kd_rate_pitch = 0.003; 
    Kp_rate_yaw   = 0.30;  Ki_rate_yaw   = 0.08;  Kd_rate_yaw   = 0.000; 

    err_roll  = p_des - pqr(1); 
    err_pitch = q_des - pqr(2); 
    err_yaw   = r_des - pqr(3); 

    % 核心保护 3: 限制积分累加幅度 (防突变量跑飞)
    roll_int  = max(-0.1, min(0.1, roll_int  + err_roll * dt)); 
    pitch_int = max(-0.1, min(0.1, pitch_int + err_pitch * dt)); 
    yaw_int   = max(-0.1, min(0.1, yaw_int   + err_yaw * dt)); 

    deriv_roll  = (err_roll  - prev_err_roll)  / dt; 
    deriv_pitch = (err_pitch - prev_err_pitch) / dt; 
    deriv_yaw   = (err_yaw   - prev_err_yaw)   / dt; 

    prev_err_roll  = err_roll; 
    prev_err_pitch = err_pitch; 
    prev_err_yaw   = err_yaw; 

    U_roll  = Kp_rate_roll  * err_roll  + Ki_rate_roll  * roll_int  + Kd_rate_roll  * deriv_roll; 
    U_pitch = Kp_rate_pitch * err_pitch + Ki_rate_pitch * pitch_int + Kd_rate_pitch * deriv_pitch; 
    U_yaw   = Kp_rate_yaw   * err_yaw   + Ki_rate_yaw   * yaw_int   + Kd_rate_yaw   * deriv_yaw; 

    % 限制控制量输出的最大权重，防止把动态范围占满
    U_roll  = max(-0.3, min(0.3, U_roll));
    U_pitch = max(-0.3, min(0.3, U_pitch));
    U_yaw   = max(-0.25, min(0.25, U_yaw));

    % 4. 混控矩阵 Mixer (Octa-Quad X 布局)
    mix = [ 
      % Thrust,   Roll,    Pitch,     Yaw
        1.0,     -0.707,   0.707,    1.0;  % Motor 1 (右前上, CCW) 
        1.0,      0.707,   0.707,   -1.0;  % Motor 2 (左前上, CW) 
        1.0,      0.707,  -0.707,    1.0;  % Motor 3 (左后上, CCW) 
        1.0,     -0.707,  -0.707,   -1.0;  % Motor 4 (右后上, CW) 
        
        1.0,     -0.707,   0.707,   -1.0;  % Motor 5 (右前下, CW) 
        1.0,      0.707,   0.707,    1.0;  % Motor 6 (左前下, CCW) 
        1.0,      0.707,  -0.707,   -1.0;  % Motor 7 (左后下, CW) 
        1.0,     -0.707,  -0.707,    1.0   % Motor 8 (右后下, CCW) 
    ]; 

    motor_cmds = mix * [T_norm; U_roll; U_pitch; U_yaw]; 

    % 5. 限幅输出
    motors = zeros(8, 1, 'uint16'); 
    for i = 1:8
        val = max(0.0, min(1.0, motor_cmds(i))); 
        motors(i) = uint16(1000.0 + val * 1000.0); 
    end
end

== matlab function air_m0c/M0A Power Measurement/M0A P Est Core ==
  data: pwm_in input; P_est output
function P_est = fcn(pwm_in)
% Estimated total shaft power proxy of all eight rotors, in W.
% UNCALIBRATED ESTIMATE (source flag 0). Mirrors the plant chart:
% omega = (pwm-1000) rad/s in [0,1000]; Q_i = C_M*omega_i^2 N*m;
% P_i = Q_i*omega_i = C_M*omega_i^3. C_M identical to plant.
pwm_min = 1000.0; pwm_max = 2000.0; omega_max = 1000.0;
C_M = 2.51e-7;
pwm_clamped = max(min(double(pwm_in), pwm_max), pwm_min);
omega = (pwm_clamped - pwm_min) / (pwm_max - pwm_min) * omega_max;
P_est = sum(C_M * omega .^ 3);
end

== matlab function air_m0c/M0A Constraint Flags/M0A Flags Core ==
  data: pwm_us input; flags output; att input; v input; P_est input; E_est input
function flags = fcn(pwm_us, att, v, P_est, E_est)
% Eight M0-A constraint flags (0/1). Thresholds are documented
% placeholders pending calibration; tune them in M0-B.
att_tol = 0.523;   % rad, 30 deg, same bound as controller phi/theta cmd
yaw_rate_tol = 1.5; % rad/s, same bound as controller r_des
speed_tol = 1.0;   % m/s, vs placeholder v_ref = 0 (no speed loop yet)
P_max = 1500.0;    % W, uncalibrated placeholder
pwm_edge = 5.0;    % us margin from the 1000/2000 rails
om = pwm_us - 1000.0;
flags = zeros(1, 8);
flags(1) = any(pwm_us <= 1000.0 + pwm_edge) || any(pwm_us >= 2000.0 - pwm_edge);
flags(2) = any(om <= pwm_edge) || any(om >= 1000.0 - pwm_edge);
flags(3) = abs(att(1)) > att_tol || abs(att(2)) > att_tol;
flags(4) = abs(att(6)) > yaw_rate_tol;
flags(5) = abs(v) > speed_tol; % v_ref = 0 placeholder until M0-B
flags(6) = P_est < 0.0 || P_est > P_max;
flags(7) = any(isnan([pwm_us(:); att(:); v; P_est; E_est]));
flags(8) = 0.0; % reserved
end

== matlab function air_m0c/M0B Reference & Safety/M0B Ref Safety Core ==
  data: optimizer_enable input; v_ref output; v_ref_manual input; v_ref_optimizer input; flags input; Ts input; status output
function [v_ref, status] = fcn(optimizer_enable, v_ref_manual, v_ref_optimizer, flags, Ts)
% M0-B reference selector + safety monitor. Safety lives here,
% never inside the future ESC core.
% status: 0 fixed baseline | 1 warm-up ramp | 2 active
%         3 frozen (hold last ref) | 4 fallback (manual ref)
persistent ref_prev hold_t clear_t fallback_latch;
if isempty(ref_prev)
    ref_prev = 0.0; hold_t = 0.0; clear_t = 0.0; fallback_latch = false;
end
v_min = 0.0; v_max = 15.0;   % v_ref range limit, m/s
rate_max = 2.0;              % v_ref rate limit, m/s per s
hold_max = 0.5;              % s frozen before fallback
clear_max = 1.5;             % s flag-free before re-engage
hard = any(flags([1 2 3 4 6 7]) > 0.5); % flag 5 logged, not gating
if optimizer_enable < 0.5
    target = v_ref_manual; status = 0.0;
    hold_t = 0.0; clear_t = 0.0; fallback_latch = false;
elseif hard
    clear_t = 0.0;
    if fallback_latch || hold_t >= hold_max
        fallback_latch = true;
        target = v_ref_manual; status = 4.0;
    else
        hold_t = hold_t + Ts;
        target = ref_prev; status = 3.0;
    end
else
    hold_t = 0.0;
    if fallback_latch
        clear_t = clear_t + Ts;
        if clear_t >= clear_max
            fallback_latch = false;
        end
        target = v_ref_manual; status = 4.0;
    else
        target = v_ref_optimizer; status = 2.0;
    end
end
target = min(v_max, max(v_min, target));
step_max = rate_max * Ts;
ramped = min(target, ref_prev + step_max);
ramped = max(ramped, ref_prev - step_max);
if status == 2.0 && abs(ramped - target) > 1e-9
    status = 1.0; % still ramping toward the selected reference
end
ref_prev = ramped;
v_ref = ramped;
end

== matlab function air_m0c/M0B Speed Controller/M0B Speed Core v2 ==
  data: enable input; pitch_cmd output; v input; ve_x input; v_ref input; Ts input; Kp input; Ki input; v_err output
function [pitch_cmd, v_err] = fcn(enable, v, ve_x, v_ref, Ts, Kp, Ki)
% M0-B speed outer loop: v_ref -> PI -> normalized pitch command
% in the chart_23 domain (theta_des = 0.523 * pitch_cmd).
% Sign convention (measured): positive pitch_cmd tilts thrust
% against +Ve_x, i.e. decelerates +x flight and accelerates -x.
% Kp (per m/s) and Ki (per m/s/s) are runtime inputs.
persistent integ prev_cmd;
if isempty(integ)
    integ = 0.0; prev_cmd = 0.0;
end
integ_max = 0.15; % integral clamp, normalized units
cmd_max = 0.40;   % |theta_des| <= 0.209 rad
rate_max = 0.25;  % normalized units per s (soft engage)
if enable < 0.5
    integ = 0.0; prev_cmd = 0.0;
    pitch_cmd = 0.0; v_err = 0.0;
    return;
end
e = v_ref - v;                   % > 0: below reference
if e < -0.10 && ve_x < 0.0
    s2 = -1.0; % too fast while flying -x: oppose the -x motion
else
    s2 = 1.0;  % default: nose-down accelerates +x (bootstrap)
end
e_eff = e * s2;
integ = min(integ_max, max(-integ_max, integ + e_eff * Ts));
cmd_raw = -(Kp * e_eff + Ki * integ);
cmd = min(cmd_max, max(-cmd_max, cmd_raw));
step_max = rate_max * Ts;
cmd = min(prev_cmd + step_max, max(prev_cmd - step_max, cmd));
prev_cmd = cmd;
pitch_cmd = cmd;
v_err = e;
end

== matlab function air_m0c/Attitude Control/quat2eul ==
  data: q input; phi output; theta output; psi output
function [phi,theta,psi] = quat2eul(q)

% Quaternion conversion to Euler angles based on the PX4 Firmware v1.6.5
% release.

phi = atan2(2*(q(1)*q(2) + q(3)* q(4)), q(1)^2 - q(2)^2 - q(3)^2 + q(4)^2);
theta = asin(-2*(q(2)*q(4) - q(1)*q(3)));
psi = atan2(2*(q(2)*q(3) + q(1)* q(4)), q(1)^2 + q(2)^2 - q(3)^2 - q(4)^2);

end
